simulink model "SVPWM_Generator"  (R2015b)
settings: Solver=ode23  StartTime=0.0  StopTime=0.05  MaxStep=1e-6  RelTol=1e-3
libraries: powerlib_meascontrol x4
settings Model: Creator=InPower 006  LastModifiedBy=InPower 006

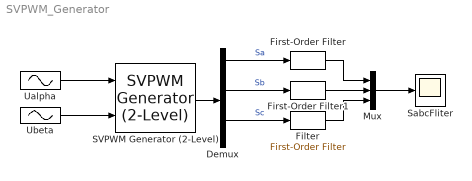
== system SVPWM_Generator ==
  Demux : Demux  Outputs=6
  Filter : powerlib_meascontrol/Filters/First-Order Filter  FilterType=Lowpass  Tc=0.0005  Ts=0  Initialize=off  Vac_Init=[0, 0, 60]  Vdc_Init=0  PlotResponse=off  FreqRange="[0,  200,  1]"
  First-Order Filter : powerlib_meascontrol/Filters/First-Order Filter  FilterType=Lowpass  Tc=0.0005  Ts=0  Initialize=off  Vac_Init=[0, 0, 60]  Vdc_Init=0  PlotResponse=off  FreqRange="[0,  200,  1]"
  First-Order Filter1 : powerlib_meascontrol/Filters/First-Order Filter  FilterType=Lowpass  Tc=0.0005  Ts=0  Initialize=off  Vac_Init=[0, 0, 60]  Vdc_Init=0  PlotResponse=off  FreqRange="[0,  200,  1]"
  Mux : Mux  Inputs=3
  SVPWM Generator (2-Level) : powerlib_meascontrol/Pulse & Signal Generators/SVPWM Generator (2-Level)  InputType=alpha-beta components  SwitchingPattern=Pattern #1  Fc=10000  ParUref=[0.8 -30 50]  Ts=0
  SabcFliter : Scope
  Ualpha : Sin  Amplitude=0.7  Frequency=2*pi*50  SampleTime=0
  Ubeta : Sin  Amplitude=0.7  Frequency=2*pi*50  Phase=pi/2  SampleTime=0
  wires:
  SVPWM Generator (2-Level)/1 -> Demux/1
  Mux/1 -> SabcFliter/1
  Demux/1 -> First-Order Filter/1  "Sa"
  Ubeta/1 -> SVPWM Generator (2-Level)/2
  Demux/5 -> Filter/1  "Sc"
  Demux/3 -> First-Order Filter1/1  "Sb"
  First-Order Filter/1 -> Mux/1
  First-Order Filter1/1 -> Mux/2
  Filter/1 -> Mux/3
  Ualpha/1 -> SVPWM Generator (2-Level)/1
